simulink model "trans001"  (R2020b)
settings: Solver=VariableStepAuto  StartTime=0.0  StopTime=10.0  RelTol=1e-3
undefined symbols (not defined in the file): L_GPP_TP1_L, L_GPP_TP1_R, L_GPP_TP2_L, L_GPP_TP2_R, L_GPP_TP4_L, L_GPP_TP4_R, L_GPP_TP5_L, L_GPP_TP5_R, L_GPP_TP7_L, L_GPP_TP7_R, L_GPP_TP8_L, L_GPP_TP8_R, L_TP2_TP3_L, L_TP2_TP3_R, L_TP5_TP6_L, L_TP5_TP6_R, Line_C, Line_HV_L, Line_HV_R, Sys_f_Hz, Sys_V_net_kV, Tr_GPP_L_pu, Tr_GPP_R_pu, Tr_GPP_Sn_VA, Tr_GPP_V_HV_kV, Tr_GPP_V_LV_kV, Tr_TP1_L_pu, Tr_TP1_R_pu, Tr_TP1_Sn_VA, Tr_TP3_L_pu, Tr_TP3_R_pu, Tr_TP3_Sn_VA, Tr_TP5_L_pu, Tr_TP5_R_pu, Tr_TP5_Sn_VA, Ts_powergui
libraries: dspstat3 x72, powerlib x46, powerlib_meascontrol x18
(part 3 of 3)

== system trans001/M_OUT_ТП8 ==
  Iptg_10 : Display
      settings: Format=bank
  PQptg_10 : Scope  NumInputPorts=2
  "Power0 (3ph, Instantaneous)" : powerlib_meascontrol/Measurements/Power (3ph, Instantaneous)
  Pptg_10 : Display
      settings: Format=bank
  Qptg_10 : Display
      settings: Format=bank
  RMS10 : dspstat3/RMS  run=off  directionMode=Each column  dimension=1  InputProcessing=Columns as channels (frame based)  reset_popup=None
  RMS3 : dspstat3/RMS  run=off  directionMode=Each column  dimension=1  InputProcessing=Columns as channels (frame based)  reset_popup=None
  RMS4 : dspstat3/RMS  run=off  directionMode=Each column  dimension=1  InputProcessing=Columns as channels (frame based)  reset_popup=None
  RMSpt_10 : dspstat3/RMS  run=off  directionMode=Each column  dimension=1  InputProcessing=Columns as channels (frame based)  reset_popup=None
  Real-Ima to Complex : RealImagToComplex
  S : Abs
  SSptg_10 : Scope
  Sptg_10 : Display
      settings: Format=bank
  Three-Phase V-I Measurementpt_10 : powerlib/Measurements/Three-Phase V-I Measurement  VoltageMeasurement=phase-to-ground  SetLabelV=off  LabelV=Vabc  Vpu=off  VpuLL=off  CurrentMeasurement=yes  SetLabelI=off  LabelI=Iabc  Ipu=off  Pbase=100e6  Vbase=500e3  OutputType=Complex  PhasorSimulation=off  PSBequivalent=0
  UIptg_10 : Scope  NumInputPorts=2
  Uptg_10 : Display
      settings: Format=bank
  a : PMIOPort  Side=Right
  b : PMIOPort  Port=2  Side=Right
  c : PMIOPort  Port=3  Side=Right
  A : PMIOPort  Port=4  Side=Left
  B : PMIOPort  Port=5  Side=Left
  C : PMIOPort  Port=6  Side=Left
  tag scope: I_ptg_10=global, P_ptg_10=global, Q_ptg_10=global, S_ptg_10=global, U_ptg_10=global
  wires:
  S/1 -> [S_ptg_10]
  Real-Ima to Complex/1 -> S/1
  [S_ptg_10] -> Sptg_10/1
  [S_ptg_10] -> SSptg_10/1
  [P_ptg_10] -> RMSpt_10/1
  RMSpt_10/1 -> Pptg_10/1
  RMS10/1 -> Qptg_10/1
  [U_ptg_10] -> RMS3/1
  RMS3/1 -> Uptg_10/1
  [P_ptg_10] -> Real-Ima to Complex/1
  [Q_ptg_10] -> RMS10/1
  [I_ptg_10] -> RMS4/1
  RMS4/1 -> Iptg_10/1
  [U_ptg_10] -> UIptg_10/1  "U"
  [P_ptg_10] -> PQptg_10/1  "P"
  [I_ptg_10] -> UIptg_10/2  "I"
  Three-Phase V-I Measurementpt_10/1 -> [U_ptg_10]
  [Q_ptg_10] -> Real-Ima to Complex/2
  Three-Phase V-I Measurementpt_10/2 -> [I_ptg_10]
  [U_ptg_10] -> "Power0 (3ph, Instantaneous)"/1
  [I_ptg_10] -> "Power0 (3ph, Instantaneous)"/2
  "Power0 (3ph, Instantaneous)"/2 -> [Q_ptg_10]
  "Power0 (3ph, Instantaneous)"/1 -> [P_ptg_10]
  [Q_ptg_10] -> PQptg_10/2  "Q"
  connections:
  Three-Phase V-I Measurementpt_10/LConn1 -- A/RConn1
  Three-Phase V-I Measurementpt_10/RConn1 -- a/RConn1
  Three-Phase V-I Measurementpt_10/LConn2 -- B/RConn1
  Three-Phase V-I Measurementpt_10/LConn3 -- C/RConn1
  Three-Phase V-I Measurementpt_10/RConn3 -- c/RConn1
  Three-Phase V-I Measurementpt_10/RConn2 -- b/RConn1
